simulink model "electromecanico_sim"  (R2022b)
settings: Solver=VariableStepAuto  StartTime=0.0  StopTime=10.0  RelTol=1e-3
values from neighbouring files (symbols this model uses):
  j = 1    [electromecanico.m]
  kb = 1    [electromecanico.m]
  kt = 1    [electromecanico.m]
  l = 1    [electrico.m]    (also in electromecanico.m = 0.5)
  r = 1    [electrico.m]    (also in electromecanico.m)
settings Model: Creator=Fran  LastModifiedBy=Fran

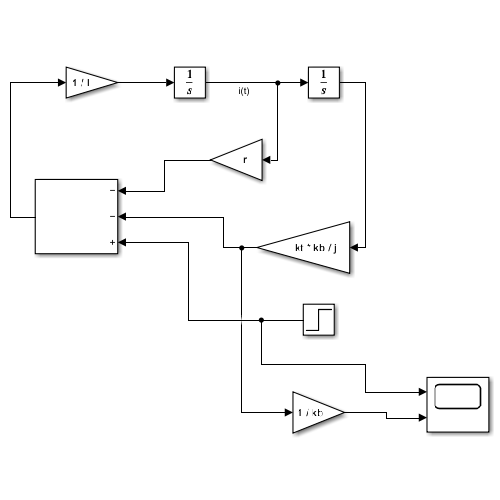
[thumbnail: Simulink's stored preview of the top-level diagram]
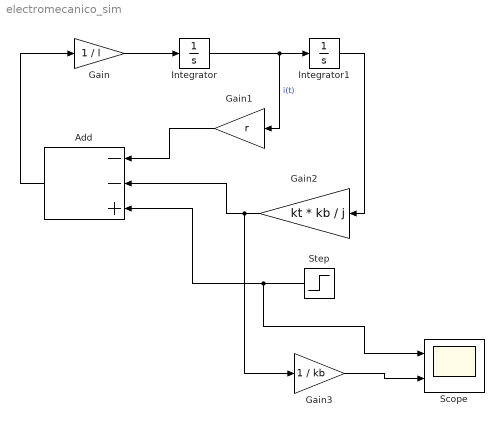
== system electromecanico_sim ==
  Add : Sum  Inputs=--+
  Gain : Gain  Gain=1 / l
  Gain1 : Gain  Gain=r
  Gain2 : Gain  Gain=kt * kb / j
  Gain3 : Gain  Gain=1 / kb
  Integrator : Integrator
  Integrator1 : Integrator
  Scope : Scope  NumInputPorts=2
  Step : Step  SampleTime=0
  wires:
  Integrator/1 -> Gain1/1, Integrator1/1  "i(t)"
  Gain/1 -> Integrator/1
  Integrator1/1 -> Gain2/1
  Step/1 -> Scope/1, Add/3
  Gain2/1 -> Gain3/1, Add/2
  Gain1/1 -> Add/1
  Add/1 -> Gain/1
  Gain3/1 -> Scope/2
